simulink model "dc_motor_model"  (R2024a)
settings: Solver=VariableStepAuto  StartTime=0.0  StopTime=30  FixedStep=0.001  RelTol=1e-3
values from neighbouring files (symbols this model uses):
  B = 1.4411e-4    (= 0.00014411)    [estimated_parameters.m]    (also in inital_parameters.m = 0.00015)
  J = 2.657e-5    (= 2.657e-05)    [estimated_parameters.m]    (also in inital_parameters.m = 9.76e-05)
  Kb = 0.0062    [estimated_parameters.m]    (also in inital_parameters.m = 0.00768)
  Km = 0.0561    [estimated_parameters.m]    (also in inital_parameters.m = 0.00768)
  L = 0.18e-3    (= 0.00018)    [estimated_parameters.m]    (also in inital_parameters.m)
  R = 4.9476    [estimated_parameters.m]    (also in inital_parameters.m = 10)
undefined symbols (not defined in the file or in its folder): tf1
settings Model: Creator=mashr  LastModifiedBy=mashr

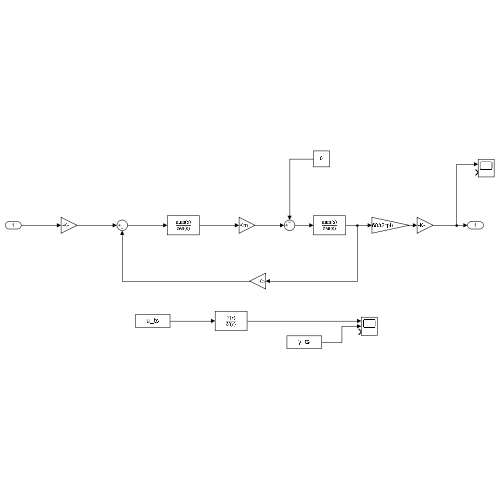
[thumbnail: Simulink's stored preview of the top-level diagram]
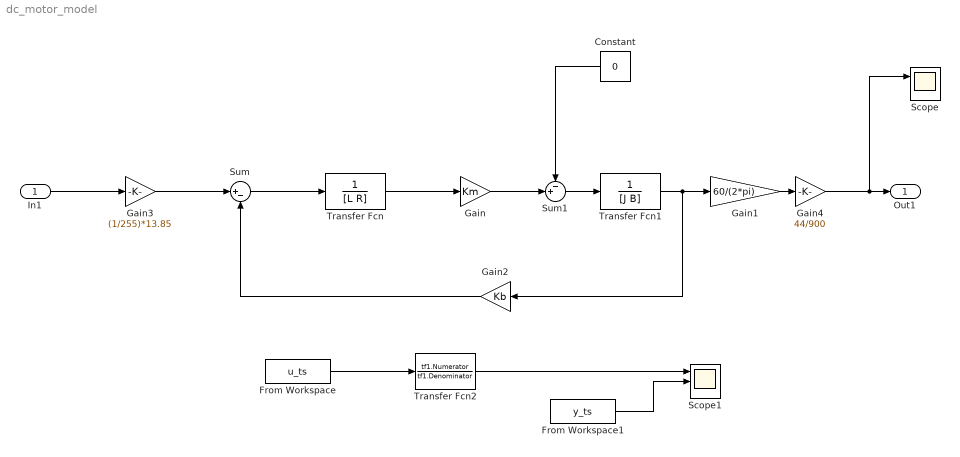
== system dc_motor_model ==
  In1 : Inport
  Constant : Constant  Value=0  SampleTime=0.01
  From Workspace : FromWorkspace  VariableName=u_ts
  From Workspace1 : FromWorkspace  VariableName=y_ts
  Gain : Gain  Gain=Km
  Gain1 : Gain  Gain=60/(2*pi)  OutDataTypeStr=double
  Gain2 : Gain  Gain=Kb
  Gain3 : Gain  Gain=(1/255)*13.85  OutDataTypeStr=double
  Gain4 : Gain  Gain=44/900  OutDataTypeStr=double
  Scope : Scope  NumInputPorts=2
  Scope1 : Scope  NumInputPorts=3
  Sum : Sum  Inputs=|+-
  Sum1 : Sum  Inputs=-+|
  Transfer Fcn : TransferFcn  Denominator=[L R]
  Transfer Fcn1 : TransferFcn  Denominator=[J B]
  Transfer Fcn2 : TransferFcn  Numerator=tf1.Numerator  Denominator=tf1.Denominator
  Out1 : Outport
  wires:
  Gain2/1 -> Sum/2
  Sum/1 -> Transfer Fcn/1
  Transfer Fcn1/1 -> Gain1/1, Gain2/1
  Gain4/1 -> Scope/1, Out1/1
  Gain/1 -> Sum1/2
  Sum1/1 -> Transfer Fcn1/1
  Constant/1 -> Sum1/1
  Transfer Fcn/1 -> Gain/1
  Gain3/1 -> Sum/1
  Gain1/1 -> Gain4/1
  In1/1 -> Gain3/1
  Transfer Fcn2/1 -> Scope1/1
  From Workspace1/1 -> Scope1/2
  From Workspace/1 -> Transfer Fcn2/1
